simulink model "driveguard_simulation"  (R2023a)
settings: Solver=VariableStepAuto  StartTime=0.0  StopTime=10.0  RelTol=1e-3
libraries: SignalEditorBlockLib x3, simulink x2
settings Model: Creator=Pulkit  LastModifiedBy=Pulkit

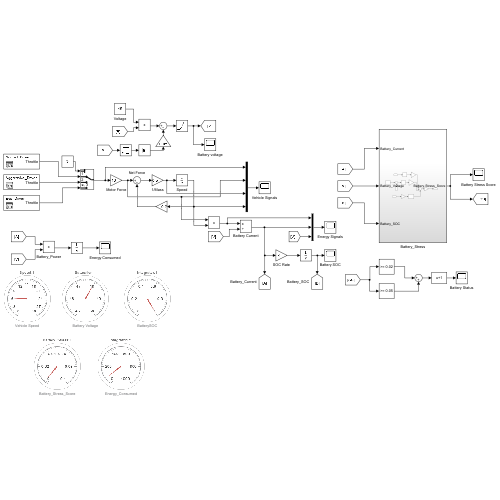
[thumbnail: Simulink's stored preview of the top-level diagram]
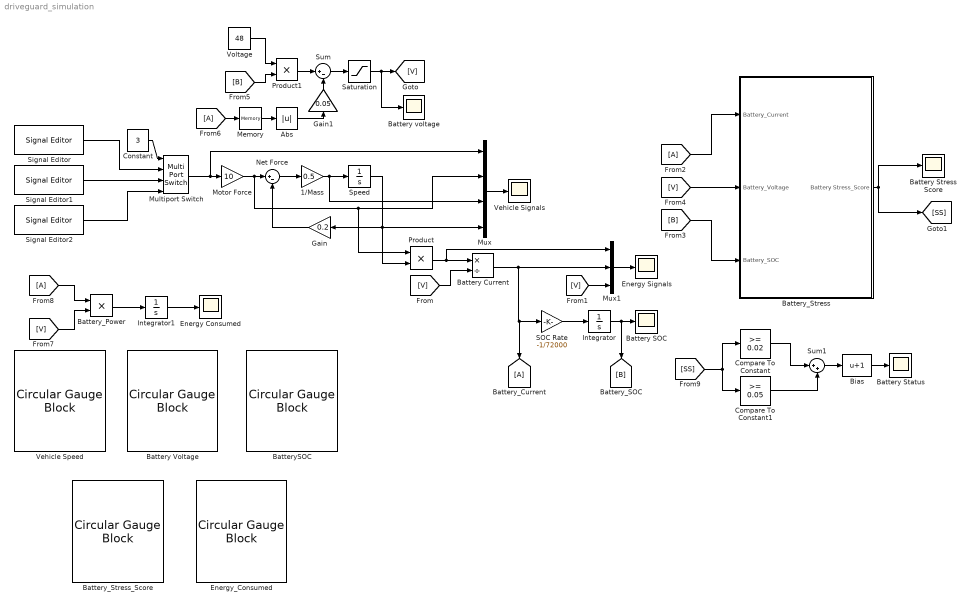
== system driveguard_simulation ==
  1/Mass : Gain  Gain=0.5
  Abs : Abs  SaturateOnIntegerOverflow=off
  Battery Current : Product  Inputs=*/
  Battery SOC : Scope
  Battery Status : Scope
  Battery Stress Score : Scope
  Battery Voltage : CircularGaugeBlock  ScaleMin=45  ScaleMax=50  TickInterval=1
  Battery voltage : Scope
  BatterySOC : CircularGaugeBlock  ScaleMax=1  TickInterval=0.2
  Battery_Current : Goto
  Battery_Power : Product
  Battery_Stress : Subsystem
  Battery_Stress_Score : CircularGaugeBlock  ScaleMax=0.1  TickInterval=0.02
  Bias : Bias  Bias=1  SaturateOnIntegerOverflow=off
  Compare To Constant : simulink/Logic and Bit Operations/Compare To Constant  relop=>=  const=0.02  OutDataTypeStr=boolean
  Compare To Constant1 : simulink/Logic and Bit Operations/Compare To Constant  relop=>=  const=0.05  OutDataTypeStr=boolean
  Constant : Constant  Value=3  SampleTime=-1
  Energy Consumed : Scope
  Energy Signals : Scope
  Energy_Consumed : CircularGaugeBlock  ScaleMax=1000  TickInterval=200
  From2 : From
  From6 : From
  From8 : From
  Gain : Gain  Gain=0.2
  Gain1 : Gain  Gain=0.05
  Integrator : Integrator  InitialCondition=1
  Integrator1 : Integrator
  Memory : Memory
  Motor Force : Gain  Gain=10
  Multiport Switch : MultiPortSwitch  SaturateOnIntegerOverflow=off  InputSameDT=off
  Mux : Mux
  Mux1 : Mux  Inputs=3
  Net Force : Sum  Inputs=|+-
  Product : Product
  Product1 : Product
  SOC Rate : Gain  Gain=-1/72000
  Saturation : Saturate  UpperLimit=100  LowerLimit=1
  Signal Editor : SignalEditorBlockLib/Signal Editor  FileName=driver_profiles.mat  ActiveScenario=Normal_Driver  ActiveSignal=Throttle  IsBus=off  OutputBusObjectStr=Bus: BusObject  SampleTime=0  Interpolate=off  ZeroCross=off  OutputAfterFinalValue=Setting to zero  Unit=inherit  PreserveSignalName=on  ApplySigPropsToAllScenarios=on
  Signal Editor1 : SignalEditorBlockLib/Signal Editor  FileName=driver_profiles.mat  ActiveScenario=Aggressive_Driver  ActiveSignal=Throttle  IsBus=off  OutputBusObjectStr=Bus: BusObject  SampleTime=0  Interpolate=off  ZeroCross=off  OutputAfterFinalValue=Setting to zero  Unit=inherit  PreserveSignalName=on  ApplySigPropsToAllScenarios=on
  Signal Editor2 : SignalEditorBlockLib/Signal Editor  FileName=driver_profiles.mat  ActiveScenario=Eco_Driver  ActiveSignal=Throttle  IsBus=off  OutputBusObjectStr=Bus: BusObject  SampleTime=0  Interpolate=off  ZeroCross=off  OutputAfterFinalValue=Setting to zero  Unit=inherit  PreserveSignalName=on  ApplySigPropsToAllScenarios=on
  Speed : Integrator
  Sum : Sum  Inputs=|+-
  Sum1 : Sum  Inputs=|++
  Vehicle Signals : Scope
  Vehicle Speed : CircularGaugeBlock  ScaleMax=30  TickInterval=3
  Voltage : Constant  Value=48
  wires:
  1/Mass/1 -> Mux/3, Speed/1
  Speed/1 -> Gain/1, Product/2, Mux/4
  Motor Force/1 -> Product/1, Mux/2, Net Force/1
  Net Force/1 -> 1/Mass/1
  Gain/1 -> Net Force/2
  Mux/1 -> Vehicle Signals/1
  Product/1 -> Battery Current/1, Mux1/1
  Battery Current/1 -> Battery_Current/1, SOC Rate/1, Mux1/2
  Mux1/1 -> Energy Signals/1
  SOC Rate/1 -> Integrator/1
  Integrator/1 -> [B], Battery SOC/1
  [V] -> Battery Current/2
  [V] -> Mux1/3
  Signal Editor/1 -> Multiport Switch/2
  Signal Editor1/1 -> Multiport Switch/3
  Signal Editor2/1 -> Multiport Switch/4
  Multiport Switch/1 -> Mux/1, Motor Force/1
  Constant/1 -> Multiport Switch/1
  From2/1 -> Battery_Stress/1(Battery_Current)
  [V] -> Battery_Stress/2(Battery_Voltage)
  [B] -> Battery_Stress/3(Battery_SOC)
  Battery_Stress/1(Battery Stress_Score) -> Battery Stress Score/1, [SS]
  [B] -> Product1/2
  Abs/1 -> Gain1/1
  Product1/1 -> Sum/1
  Gain1/1 -> Sum/2
  From6/1 -> Memory/1
  Memory/1 -> Abs/1
  Voltage/1 -> Product1/1
  Sum/1 -> Saturation/1
  Saturation/1 -> Battery voltage/1, [V]
  From8/1 -> Battery_Power/1
  [V] -> Battery_Power/2
  Battery_Power/1 -> Integrator1/1
  Integrator1/1 -> Energy Consumed/1
  [SS] -> Compare To Constant1/1, Compare To Constant/1
  Compare To Constant/1 -> Sum1/1
  Compare To Constant1/1 -> Sum1/2
  Sum1/1 -> Bias/1
  Bias/1 -> Battery Status/1

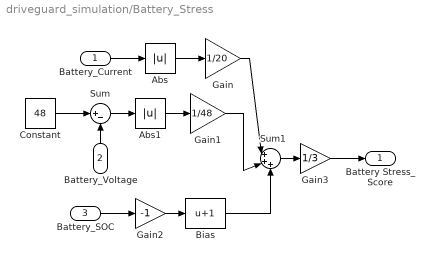
== system driveguard_simulation/Battery_Stress ==
  Battery_Current : Inport
  Battery_Voltage : Inport  Port=2
  Battery_SOC : Inport  Port=3
  Abs : Abs  SaturateOnIntegerOverflow=off
  Abs1 : Abs  SaturateOnIntegerOverflow=off
  Bias : Bias  Bias=1  SaturateOnIntegerOverflow=off
  Constant : Constant  Value=48
  Gain : Gain  Gain=1/20
  Gain1 : Gain  Gain=1/48
  Gain2 : Gain  Gain=-1
  Gain3 : Gain  Gain=1/3
  Sum : Sum  Inputs=|+-
  Sum1 : Sum  Inputs=|+++
  Battery Stress_Score : Outport
  wires:
  Battery_Current/1 -> Abs/1
  Abs/1 -> Gain/1
  Battery_Voltage/1 -> Sum/2
  Constant/1 -> Sum/1
  Battery_SOC/1 -> Gain2/1
  Gain2/1 -> Bias/1
  Gain/1 -> Sum1/1
  Gain1/1 -> Sum1/2
  Bias/1 -> Sum1/3
  Sum1/1 -> Gain3/1
  Gain3/1 -> Battery Stress_Score/1
  Sum/1 -> Abs1/1
  Abs1/1 -> Gain1/1
